simulink model "Simple_Hinf"  (R2019a)
settings: Solver=VariableStepAuto  StartTime=0.0  StopTime=10.0  RelTol=1e-3
settings Model: Creator=martin  LastModifiedBy=martin

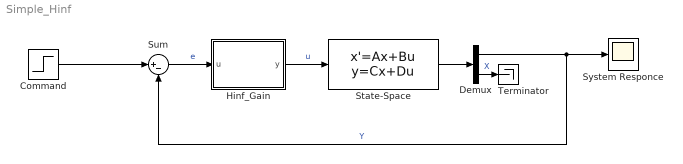
== system Simple_Hinf ==
  Command : Step  SampleTime=0
  Demux : Demux  Outputs=2
  Hinf_Gain : MATLAB Function  TreatAsAtomicUnit=on
  State-Space : StateSpace  InitialCondition=0
  Sum : Sum  Inputs=|+-
  System Responce : Scope
  Terminator : Terminator
  wires:
  State-Space/1 -> Demux/1
  Demux/1 -> Sum/2, System Responce/1  "Y"
  Demux/2 -> Terminator/1  "X"
  Sum/1 -> Hinf_Gain/1(u)  "e"
  Command/1 -> Sum/1
  Hinf_Gain/1(y) -> State-Space/1  "u"

== matlab function Simple_Hinf/Hinf_Gain ==
  data: u input; y output
function y = fcn(u)

y = u;
